simulink model "scheme_batch_op_regulation"  (R2025a)
settings: Solver=ode3  StartTime=0.0  StopTime=40  FixedStep=dt  RelTol=1e-3
values from neighbouring files (symbols this model uses):
  dt = 0.0001    [Planning_w_Adaptive.m]    (also in runBatchTests.m = 0.0005; tune_mrac_params.m = 0.01)
  map_scale = 0.5    [Planning_w_Adaptive.m]    (also in tune_mrac_params.m)
  N = -1 / (C_output_phi * inv(Am) * B)    [Planning_w_Adaptive.m]    (also in tune_mrac_params.m)
  op_space_pose_trajectory = zeros(4, 4, num_points)    [runBatchTests.m]
  waypoints = pathObj.States(:, 1:2)    [Planning_w_Adaptive.m]    (also in tune_mrac_params.m)
  x0 = zeros(10, 1)    [LQR_Control_generated.m]    (also in PID_LQR_PI_Loop.m = zeros(14, 1); Planning_w_Adaptive.m)
undefined symbols (not defined in the file or in its folder): control_params, initial_positions_rad, manipulator_time_vector, p, X, Y, Z
libraries: sm_lib x179, nesl_utility x28, fl_lib x3
(part 5 of 5)

== matlab function scheme_batch_op_regulation/MATLAB Function2 ==
  data: x input; h_base output; p parameter
function h_base = calculate_base_height(x, p)
% =========================================================================
% CALCULATE_BASE_HEIGHT
%
% This function calculates the instantaneous height of the manipulator base
% relative to the ground, accounting for the ballbot's tilt angles.
%
% INPUTS:
%   x   (vector): The state vector of the ballbot. It is assumed that:
%                 x(1) = theta_x (roll angle) [rad]
%                 x(2) = theta_y (pitch angle) [rad]
%   p   (struct): The system parameters struct, which must contain:
%                 p.h_U = height of the manipulator base when upright [m]
%                 p.r_S = radius of the spherical wheel [m]
%
% OUTPUT:
%   h_base (scalar): The calculated instantaneous height of the base [m]
% =========================================================================

    % --- Step 1: Unpack the Tilt Angles from the State Vector ---
    % Get the roll (transversal plane) and pitch (sagittal plane) angles.
    theta_x = x(1);
    theta_y = x(2);

    % --- Step 2: Calculate the Virtual "Pendulum" Length ---
    % This is the distance from the center of the sphere to the manipulator base.
    L = p.h_U - p.r_S;

    % --- Step 3: Calculate the Instantaneous Height ---
    % The final height is the sphere's radius plus the vertical component
    % of the tilted pendulum length.
    h_base = p.r_S + L * cos(theta_x) * cos(theta_y);

end

== matlab function scheme_batch_op_regulation/PID velocity Generator ==
  settings: updateMethod=DISCRETE
  data: x input; phi_dot_c output; waypoints input; p parameter; dt parameter; control_params parameter; map_scale parameter; simtime input
function phi_dot_c  = calculate_velocity_command_PID(x, waypoints, p, dt, control_params, map_scale, simtime)
% =========================================================================
% CALCULATE_VELOCITY_COMMAND_PID (v3 - With Conditional Derivative)
%
% This version includes checks to disable the derivative (D) action:
% 1. At the start of the simulation (t < 0.5s).
% 2. For the single time step when the target waypoint is switched.
% =========================================================================

persistent current_waypoint_idx integral_error prev_error;

if isempty(current_waypoint_idx)
    current_waypoint_idx = 1;
    integral_error = [0; 0];
    prev_error = [0; 0];
end

% --- WAYPOINT NAVIGATION LOGIC ---
%waypoint_has_switched = false; % <-- ADDED: Flag to detect a waypoint switch.
waypoint_reach_threshold = 0.15 * map_scale;

if current_waypoint_idx > size(waypoints, 1)
    current_waypoint_idx = size(waypoints, 1);
end

p_target = waypoints(current_waypoint_idx, :)';
p_current = [p.r_S * x(5); -p.r_S * x(4)];

distance_to_target = norm(p_current - p_target);
if (distance_to_target < waypoint_reach_threshold) && (current_waypoint_idx < size(waypoints, 1))
    current_waypoint_idx = current_waypoint_idx + 1;
    integral_error = [0; 0];
    %waypoint_has_switched = true; % <-- ADDED: Set flag to true for one cycle.
end

% --- PID CONTROLLER CALCULATION ---
position_error = p_target - p_current;
integral_error = integral_error + position_error * dt;
%derivative_error = (position_error - prev_error) / dt;

% Calculate PI terms first. The output is a linear velocity command (v_cmd).
P_term = control_params.Kp_pos .* position_error;
%I_term = control_params.Ki_pos .* integral_error;
v_cmd = P_term; %+ I_term;

% <-- MODIFIED: Conditionally add the Derivative term -->
% The D_term is added ONLY if the simulation has run for more than 0.5s
% AND the waypoint has NOT just switched in this very time step.
% D_term = control_params.Kd_pos .* derivative_error;
% if simtime > 0.5 && ~waypoint_has_switched
%     v_cmd = v_cmd + D_term;
% end

% Update state for the next iteration
prev_error = position_error;

% <-- SATURATE VELOCITY COMMAND -->
% Convert it to the corresponding maximum linear velocity (m/s)
max_v_cmd =0.3;

% Check if the magnitude of the command vector exceeds the limit
v_cmd_magnitude = norm(v_cmd);
if v_cmd_magnitude > max_v_cmd
    % Scale the vector down to the maximum magnitude while preserving its direction
    v_cmd = v_cmd / v_cmd_magnitude * max_v_cmd;
end

% --- FORMAT OUTPUT ---
% Convert the final linear velocity command (v_cmd in m/s) to an
% angular velocity command (phi_dot_c in rad/s).
phi_dot_c = [v_cmd(1) / p.r_S; -v_cmd(2) / p.r_S];

end
